simulink model "VS_Plausability"  (R2024b)
settings: Solver=VariableStepAuto  StartTime=0.0  StopTime=16  RelTol=1e-3
libraries: simulink x1
settings Model: Creator=Michele  LastModifiedBy=Michele
settings ConfigComp: CovEnable=on  RecordCoverage=on  CovMetricSettings=dcmwe  CovModelRefEnable=on

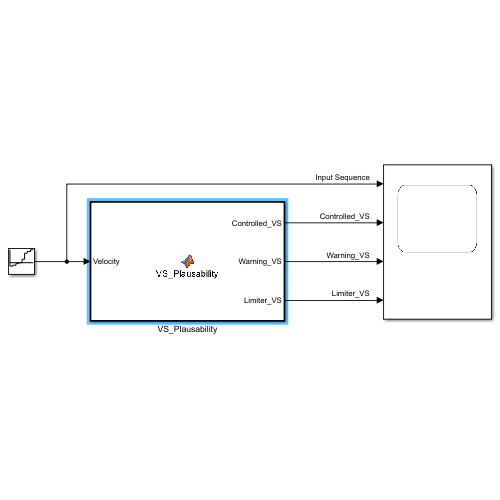
[thumbnail: Simulink's stored preview of the top-level diagram]
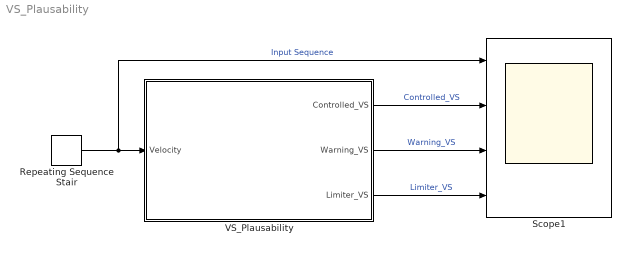
== system VS_Plausability ==
  Repeating Sequence Stair : simulink/Sources/Repeating Sequence Stair  OutValues="[-80 -80 -60 -60  -30 -30 0 0 80 80 200 200 240 240 280  280 ].'"  tsamp=1  OutMin=[]  OutMax=[]  OutDataTypeStr=single  OutputDataTypeScalingMode=single  OutDataType=Enum: TransmissionState  ConRadixGroup=Best Precision: Vector-wise  OutScaling=[]
  Scope1 : Scope  NumInputPorts=4
  VS_Plausability : MATLAB Function  TreatAsAtomicUnit=on
  wires:
  VS_Plausability/3(Limiter_VS) -> Scope1/4  "Limiter_VS"
  VS_Plausability/1(Controlled_VS) -> Scope1/2  "Controlled_VS"
  VS_Plausability/2(Warning_VS) -> Scope1/3  "Warning_VS"
  Repeating Sequence Stair/1 -> Scope1/1, VS_Plausability/1(Velocity)  "Input Sequence"

== matlab function VS_Plausability/VS_Plausability ==
  data: Velocity input single; Controlled_VS output single; Warning_VS output Enum: WarningType; Limiter_VS output boolean
function [Controlled_VS,Warning_VS,Limiter_VS] = VS_Plausability(Velocity)

Controlled_VS = single(Velocity);
Warning_VS =  WarningType(0);
Limiter_VS = boolean(0);

if (Velocity > 240 || Velocity < -60)

    Warning_VS =  WarningType(1);
    Limiter_VS = boolean(1);

end
